simulink model "position_control_design"  (R2018b)
settings: Solver=VariableStepAuto  StartTime=0.0  StopTime=5  RelTol=1e-3
settings Model: Creator=Tyler  LastModifiedBy=Tyler

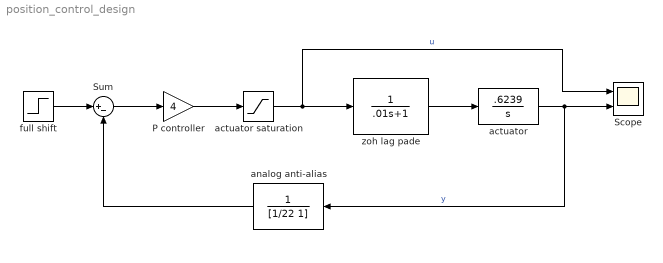
== system position_control_design ==
  P controller : Gain  Gain=4
  Scope : Scope  NumInputPorts=2
  Sum : Sum  Inputs=|+-
  actuator : TransferFcn  Numerator=[.6239]  Denominator=[1 0]
  actuator saturation : Saturate  UpperLimit=500  LowerLimit=-500
  analog anti-alias : TransferFcn  Denominator=[1/22 1]
  full shift : Step  Time=0  After=615  SampleTime=0
  zoh lag pade : TransferFcn  Denominator=[.01 1]
  wires:
  full shift/1 -> Sum/1
  Sum/1 -> P controller/1
  actuator saturation/1 -> zoh lag pade/1, Scope/1  "u"
  actuator/1 -> Scope/2, analog anti-alias/1  "y"
  zoh lag pade/1 -> actuator/1
  analog anti-alias/1 -> Sum/2
  P controller/1 -> actuator saturation/1
